simulink library "UseControlValueIfFaulty"  (R2019b)
settings: Solver=VariableStepAuto  StartTime=0.0  StopTime=10.0  RelTol=1e-3
settings Model: Creator=hp  LastModifiedBy=hp

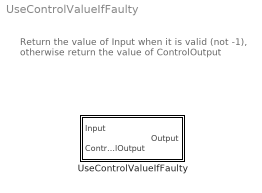
== system UseControlValueIfFaulty ==
  note: Return the value of Input when it is valid (not -1),
      | otherwise return the value of ControlOutput
  UseControlValueIfFaulty : Subsystem

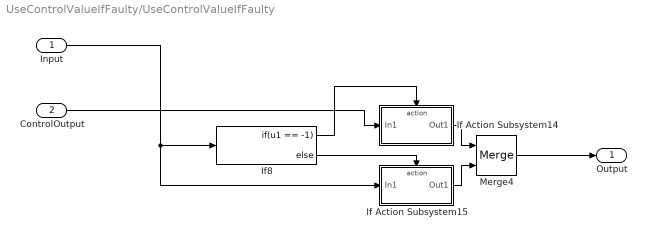
== system UseControlValueIfFaulty/UseControlValueIfFaulty ==
  Input : Inport
  ControlOutput : Inport  Port=2
  If Action Subsystem14 : Subsystem  TreatAsAtomicUnit=on
  If Action Subsystem15 : Subsystem  TreatAsAtomicUnit=on
  If8 : If  IfExpression=u1 == -1
  Merge4 : Merge
  Output : Outport
  wires:
  If8/1 -> If Action Subsystem14/Action
  ControlOutput/1 -> If Action Subsystem14/1(In1)
  If Action Subsystem15/1(Out1) -> Merge4/2
  If8/2 -> If Action Subsystem15/Action
  If Action Subsystem14/1(Out1) -> Merge4/1
  Input/1 -> If8/1, If Action Subsystem15/1(In1)
  Merge4/1 -> Output/1

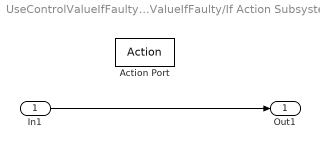
== system UseControlValueIfFaulty/UseControlValueIfFaulty/If Action Subsystem14 ==
  In1 : Inport
  Action Port : ActionPort  ActionPortLabel=if(u1 == -1)
  Out1 : Outport
  wires:
  In1/1 -> Out1/1

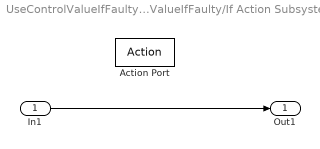
== system UseControlValueIfFaulty/UseControlValueIfFaulty/If Action Subsystem15 ==
  In1 : Inport
  Action Port : ActionPort  ActionPortLabel=else
  Out1 : Outport
  wires:
  In1/1 -> Out1/1
